simulink model "Separate_Excited_DC_Motor"  (R2021a)
settings: Solver=VariableStepAuto  StartTime=0.0  StopTime=1  RelTol=1e-3
settings Model: Creator=SA  LastModifiedBy=SA

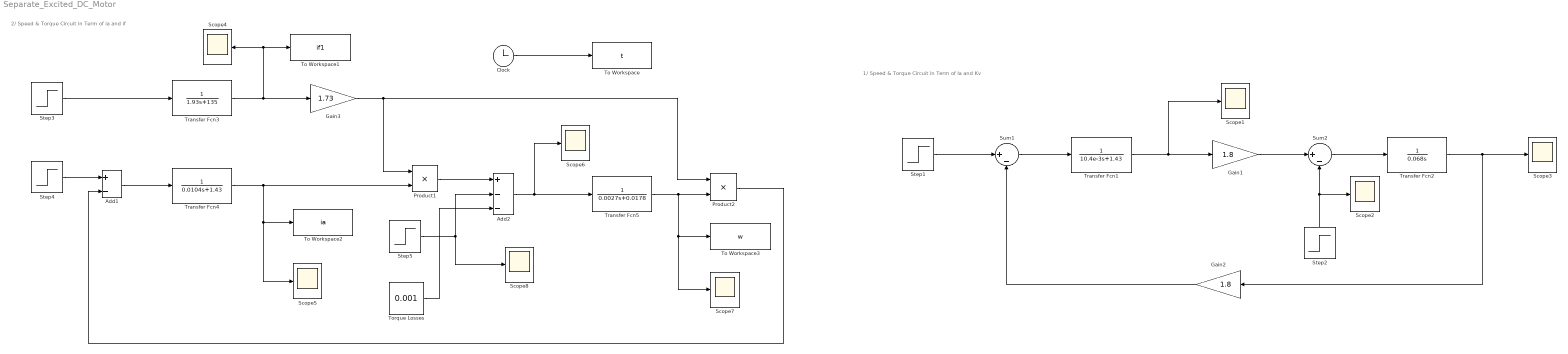
== system Separate_Excited_DC_Motor ==
  note: 2/ Speed & Torque Circuit in Term of ia and if
  note: 1/ Speed & Torque Circuit in Term of Ia and Kv
  Add1 : Sum  Inputs=+-
  Add2 : Sum  Inputs=+--
  Clock : Clock
  Gain1 : Gain  Gain=1.8
  Gain2 : Gain  Gain=1.8
  Gain3 : Gain  Gain=1.73
  Product1 : Product
  Product2 : Product
  Scope{1..8} (8 alike) : Scope
  Step1 : Step  Time=0  After=240  SampleTime=0
  Step2 : Step  Time=0.1  After=-302  SampleTime=0
  Step3 : Step  Time=0  After=115  SampleTime=0
  Step4 : Step  Time=0  After=240  SampleTime=0
  Step5 : Step  Time=0.1  After=-1000  SampleTime=0
  Sum1 : Sum  Inputs=|+-
  Sum2 : Sum  Inputs=|+-
  To Workspace : ToWorkspace  VariableName=t  SaveFormat=Timeseries  SampleTime=-1
  To Workspace1 : ToWorkspace  VariableName=if1  SaveFormat=Timeseries  SampleTime=-1
  To Workspace2 : ToWorkspace  VariableName=ia  SaveFormat=Timeseries  SampleTime=-1
  To Workspace3 : ToWorkspace  VariableName=w  SaveFormat=Timeseries  SampleTime=-1
  Torque Losses : Constant  Value=0.001
  Transfer Fcn1 : TransferFcn  Denominator=[10.4e-3 1.43]
  Transfer Fcn2 : TransferFcn  Denominator=[0.068 0]
  Transfer Fcn3 : TransferFcn  Denominator=[1.93 135]
  Transfer Fcn4 : TransferFcn  Denominator=[0.0104 1.43]
  Transfer Fcn5 : TransferFcn  Denominator=[0.0027 0.0178]
  wires:
  Step1/1 -> Sum1/1
  Sum1/1 -> Transfer Fcn1/1
  Transfer Fcn1/1 -> Gain1/1, Scope1/1
  Gain1/1 -> Sum2/1
  Step2/1 -> Scope2/1, Sum2/2
  Sum2/1 -> Transfer Fcn2/1
  Transfer Fcn2/1 -> Scope3/1, Gain2/1
  Gain2/1 -> Sum1/2
  Add1/1 -> Transfer Fcn4/1
  Transfer Fcn4/1 -> Scope5/1, To Workspace2/1, Product1/2
  Product1/1 -> Add2/1
  Gain3/1 -> Product1/1, Product2/1
  Transfer Fcn3/1 -> To Workspace1/1, Scope4/1, Gain3/1
  Step3/1 -> Transfer Fcn3/1
  Step4/1 -> Add1/1
  Step5/1 -> Scope8/1, Add2/2
  Torque Losses/1 -> Add2/3
  Add2/1 -> Scope6/1, Transfer Fcn5/1
  Transfer Fcn5/1 -> Scope7/1, To Workspace3/1, Product2/2
  Product2/1 -> Add1/2
  Clock/1 -> To Workspace/1
